simulink model "W1Q8"  (R2020a)
settings: Solver=VariableStepAuto  StartTime=0.0  StopTime=10.0  RelTol=1e-3
settings Model: Creator=Vinayak  LastModifiedBy=Vinayak

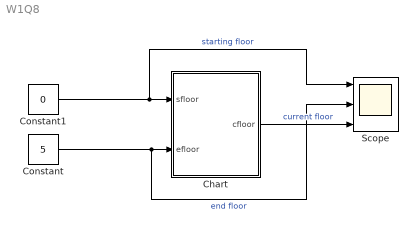
== system W1Q8 ==
  Chart : Stateflow chart  TreatAsAtomicUnit=on
  Constant : Constant  Value=5
  Constant1 : Constant  Value=0
  Scope : Scope  NumInputPorts=3
  wires:
  Constant/1 -> Scope/2, Chart/2(efloor)  "end floor"
  Constant1/1 -> Scope/1, Chart/1(sfloor)  "starting floor"
  Chart/1(cfloor) -> Scope/3  "current floor"

== stateflow chart W1Q8/Chart ==
  settings: sampleTime=0.001
  state Floor5
    entry:
    during:
    cfloor=5;
  state Floor4
    entry:
    during:
    cfloor=4;
  state Floor3
    entry:
    during:
    cfloor=3;
  state Floor2
    entry:
    during:
    cfloor=2;
  state Floor1
    entry:
    during:
    cfloor=1;
  state Floor0
    entry:
    during:
    cfloor=1;
  state Start
    entry:
    x=sfloor;
    y=x;
    during:
    cfloor=0;
  Floor5 -> Floor5 [order 2] : after(3,sec)[efloor==5]
  Start -> Floor5 [order 5] : [y==5]
  Floor4 -> Floor5 [order 1] : after(3,sec)[efloor~=4&&efloor>4]
  Floor5 -> Floor4 [order 1] : after(3,sec)[efloor~=5&&efloor<5]
  Floor4 -> Floor4 [order 3] : [efloor==4]
  Start -> Floor4 [order 4] : [y==4]
  Floor3 -> Floor4 [order 1] : after(3,sec)[efloor~=3&&efloor>3]
  Floor4 -> Floor3 [order 2] : after(3,sec)[efloor~=4&&efloor<4]
  Floor3 -> Floor3 [order 3] : [efloor==3]
  Start -> Floor3 [order 3] : [y==3]
  Floor2 -> Floor3 [order 1] : after(3,sec)[efloor~=2&&efloor>2]
  Floor3 -> Floor2 [order 2] : after(3,sec)[efloor~=3&&efloor<3]
  Start -> Floor2 [order 2] : [y==2]
  Start -> Floor1 [order 1] : [y==1]
  Floor2 -> Floor2 [order 3] : [efloor==2]
  Floor1 -> Floor2 [order 1] : after(3,sec)[efloor~=1&&efloor>1]
  Floor2 -> Floor1 [order 2] : after(3,sec)[efloor~=2&&efloor<2]
  Floor1 -> Floor1 [order 2] : [efloor==1]
  Floor0 -> Floor1 [order 1] : after(3,sec)[efloor~=0&&efloor>0]
  Floor1 -> Floor0 [order 3] : after(3,sec)[efloor~=1&&efloor<1]
  Floor0 -> Floor0 [order 2] : [efloor==0&&efloor==sfloor]
  Start -> Floor0 [order 6] : [y==0]
  (default) -> Start
  data: sfloor input; efloor input; cfloor output; x local; y local
